simulink model "case6"  (R2024b)
settings: Solver=FixedStepAuto  StartTime=0  StopTime=1  FixedStep=1e-7  RelTol=1e-3
values from neighbouring files (symbols this model uses):
  SG_D_1_D = 0.01056    [IEEE9_case_parameters.m]    (also in case1_parameters.m; case2_parameters.m; case3_parameters.m; case4_parameters.m)
  SG_D_1_EnableSaturation = 0    [IEEE9_case_parameters.m]    (also in case1_parameters.m; case2_parameters.m; case3_parameters.m; case4_parameters.m)
  SG_D_1_f0 = 60    [IEEE9_case_parameters.m]    (also in case1_parameters.m; case2_parameters.m; case3_parameters.m; case4_parameters.m)
  SG_D_1_H = 7.5    [IEEE9_case_parameters.m]    (also in case1_parameters.m; case2_parameters.m; case3_parameters.m; case4_parameters.m)
  SG_D_1_K_A = 20    [IEEE9_case_parameters.m]    (also in case1_parameters.m; case2_parameters.m; case3_parameters.m; case4_parameters.m)
  SG_D_1_K_E = 1.000000e+1    (= 10)    [IEEE9_case_parameters.m]    (also in case1_parameters.m; case2_parameters.m; case3_parameters.m; case4_parameters.m)
  SG_D_1_K_F = 2.363    [IEEE9_case_parameters.m]    (also in case1_parameters.m; case2_parameters.m; case3_parameters.m; case4_parameters.m)
  SG_D_1_K_s = 0.5    [IEEE9_case_parameters.m]    (also in case1_parameters.m = 5; case2_parameters.m = 5; case3_parameters.m = 5; case4_parameters.m = 5)
  SG_D_1_R_a = 0.001088    [IEEE9_case_parameters.m]    (also in case1_parameters.m; case2_parameters.m; case3_parameters.m; case4_parameters.m)
  SG_D_1_S_A = 1    [IEEE9_case_parameters.m]    (also in case1_parameters.m; case2_parameters.m; case3_parameters.m; case4_parameters.m)
  SG_D_1_S_B = 0.103    [IEEE9_case_parameters.m]    (also in case1_parameters.m; case2_parameters.m; case3_parameters.m; case4_parameters.m)
  SG_D_1_S_N = 10.659857    [IEEE9_case_parameters.m]    (also in case1_parameters.m; case2_parameters.m; case3_parameters.m; case4_parameters.m)
  SG_D_1_SpeedPara = 200    [IEEE9_case_parameters.m]    (also in case1_parameters.m; case2_parameters.m; case3_parameters.m; case4_parameters.m)
  SG_D_1_T_0 = 0.720173    [IEEE9_case_parameters.m]    (also in case1_parameters.m = 0.755522; case2_parameters.m = 0.808931; case3_parameters.m = 0.869402; case4_parameters.m = 0.729316)
  SG_D_1_T_1 = 0.3    [IEEE9_case_parameters.m]    (also in case1_parameters.m; case2_parameters.m; case3_parameters.m; case4_parameters.m)
  SG_D_1_T_2 = 0.05    [IEEE9_case_parameters.m]    (also in case1_parameters.m; case2_parameters.m; case3_parameters.m; case4_parameters.m)
  SG_D_1_T_3 = 0.02    [IEEE9_case_parameters.m]    (also in case1_parameters.m; case2_parameters.m; case3_parameters.m; case4_parameters.m)
  SG_D_1_T_4 = 0.005    [IEEE9_case_parameters.m]    (also in case1_parameters.m; case2_parameters.m; case3_parameters.m; case4_parameters.m)
  SG_D_1_T_A = 0.02    [IEEE9_case_parameters.m]    (also in case1_parameters.m; case2_parameters.m; case3_parameters.m; case4_parameters.m)
  SG_D_1_T_dd = 8.000000e+0    (= 8)    [IEEE9_case_parameters.m]    (also in case1_parameters.m; case2_parameters.m; case3_parameters.m; case4_parameters.m)
  SG_D_1_T_ddd = 0.04    [IEEE9_case_parameters.m]    (also in case1_parameters.m; case2_parameters.m; case3_parameters.m; case4_parameters.m)
  SG_D_1_T_E = 0.314    [IEEE9_case_parameters.m]    (also in case1_parameters.m; case2_parameters.m; case3_parameters.m; case4_parameters.m)
  SG_D_1_T_F = 0.35    [IEEE9_case_parameters.m]    (also in case1_parameters.m; case2_parameters.m; case3_parameters.m; case4_parameters.m)
  SG_D_1_T_qd = 0.8    [IEEE9_case_parameters.m]    (also in case1_parameters.m; case2_parameters.m; case3_parameters.m; case4_parameters.m)
  SG_D_1_T_qdd = 0.02    [IEEE9_case_parameters.m]    (also in case1_parameters.m; case2_parameters.m; case3_parameters.m; case4_parameters.m)
  SG_D_1_T_speed = 0.1    [IEEE9_case_parameters.m]    (also in case1_parameters.m = 200; case2_parameters.m = 200; case3_parameters.m = 200; case4_parameters.m = 200)
  SG_D_1_T_w = 0.5    [IEEE9_case_parameters.m]    (also in case1_parameters.m; case2_parameters.m; case3_parameters.m; case4_parameters.m)
  SG_D_1_V_ref = 1.990276    [IEEE9_case_parameters.m]    (also in case1_parameters.m = 2.042296; case2_parameters.m = 2.051388; case3_parameters.m = 2.089584; case4_parameters.m = 2.01845)
  SG_D_1_w_ref = 376.991118    [IEEE9_case_parameters.m]    (also in case1_parameters.m; case2_parameters.m; case3_parameters.m; case4_parameters.m)
  SG_D_1_wb = 6.000000e+1    (= 60)    [IEEE9_case_parameters.m]    (also in case1_parameters.m; case2_parameters.m; case3_parameters.m; case4_parameters.m)
  SG_D_1_x_d = 1.9    [IEEE9_case_parameters.m]    (also in case1_parameters.m; case2_parameters.m; case3_parameters.m; case4_parameters.m)
  SG_D_1_x_dd = 0.302    [IEEE9_case_parameters.m]    (also in case1_parameters.m; case2_parameters.m; case3_parameters.m; case4_parameters.m)
  SG_D_1_x_ddd = 0.204    [IEEE9_case_parameters.m]    (also in case1_parameters.m; case2_parameters.m; case3_parameters.m; case4_parameters.m)
  SG_D_1_x_l = 0.05    [IEEE9_case_parameters.m]    (also in case1_parameters.m; case2_parameters.m; case3_parameters.m; case4_parameters.m)
  SG_D_1_x_q = 1.3    [IEEE9_case_parameters.m]    (also in case1_parameters.m; case2_parameters.m; case3_parameters.m; case4_parameters.m)
  SG_D_1_x_qd = 0.5    [IEEE9_case_parameters.m]    (also in case1_parameters.m; case2_parameters.m; case3_parameters.m; case4_parameters.m)
  SG_D_1_x_qdd = 0.3    [IEEE9_case_parameters.m]    (also in case1_parameters.m; case2_parameters.m; case3_parameters.m; case4_parameters.m)
  SG_D_2_D = 0.02    [IEEE9_case_parameters.m]    (also in case1_parameters.m; case2_parameters.m; case3_parameters.m; case4_parameters.m)
  SG_D_2_EnableSaturation = 0    [IEEE9_case_parameters.m]    (also in case1_parameters.m; case2_parameters.m; case3_parameters.m; case4_parameters.m)
  SG_D_2_f0 = 60    [IEEE9_case_parameters.m]    (also in case1_parameters.m; case2_parameters.m; case3_parameters.m; case4_parameters.m)
  SG_D_2_H = 8.000000e+0    (= 8)    [IEEE9_case_parameters.m]    (also in case1_parameters.m; case2_parameters.m; case3_parameters.m; case4_parameters.m)
  SG_D_2_K_A = 20    [IEEE9_case_parameters.m]    (also in case1_parameters.m; case2_parameters.m; case3_parameters.m; case4_parameters.m)
  SG_D_2_K_E = 1.000000e+1    (= 10)    [IEEE9_case_parameters.m]    (also in case1_parameters.m; case2_parameters.m; case3_parameters.m; case4_parameters.m)
  SG_D_2_K_F = 2.363    [IEEE9_case_parameters.m]    (also in case1_parameters.m; case2_parameters.m; case3_parameters.m; case4_parameters.m)
  SG_D_2_K_s = 0.5    [IEEE9_case_parameters.m]    (also in case1_parameters.m = 4; case2_parameters.m = 4; case3_parameters.m = 4; case4_parameters.m = 4)
  SG_D_2_R_a = 0.001088    [IEEE9_case_parameters.m]    (also in case1_parameters.m; case2_parameters.m; case3_parameters.m; case4_parameters.m)
  SG_D_2_S_A = 1    [IEEE9_case_parameters.m]    (also in case1_parameters.m; case2_parameters.m; case3_parameters.m; case4_parameters.m)
  SG_D_2_S_B = 0.103    [IEEE9_case_parameters.m]    (also in case1_parameters.m; case2_parameters.m; case3_parameters.m; case4_parameters.m)
  SG_D_2_S_N = 10.659857    [IEEE9_case_parameters.m]    (also in case1_parameters.m; case2_parameters.m; case3_parameters.m; case4_parameters.m)
  SG_D_2_SpeedPara = 200    [IEEE9_case_parameters.m]    (also in case1_parameters.m; case2_parameters.m; case3_parameters.m; case4_parameters.m)
  SG_D_2_T_0 = 1.632913    [IEEE9_case_parameters.m]    (also in case1_parameters.m = 1.632925; case2_parameters.m = 1.632915; case3_parameters.m = 1.632914; case4_parameters.m = 1.632927)
  SG_D_2_T_1 = 0.2    [IEEE9_case_parameters.m]    (also in case1_parameters.m; case2_parameters.m; case3_parameters.m; case4_parameters.m)
  SG_D_2_T_2 = 0.05    [IEEE9_case_parameters.m]    (also in case1_parameters.m; case2_parameters.m; case3_parameters.m; case4_parameters.m)
  SG_D_2_T_3 = 0.02    [IEEE9_case_parameters.m]    (also in case1_parameters.m; case2_parameters.m; case3_parameters.m; case4_parameters.m)
  SG_D_2_T_4 = 0.005    [IEEE9_case_parameters.m]    (also in case1_parameters.m; case2_parameters.m; case3_parameters.m; case4_parameters.m)
  SG_D_2_T_A = 0.02    [IEEE9_case_parameters.m]    (also in case1_parameters.m; case2_parameters.m; case3_parameters.m; case4_parameters.m)
  SG_D_2_T_dd = 7.9    [IEEE9_case_parameters.m]    (also in case1_parameters.m; case2_parameters.m; case3_parameters.m; case4_parameters.m)
  SG_D_2_T_ddd = 0.04    [IEEE9_case_parameters.m]    (also in case1_parameters.m; case2_parameters.m; case3_parameters.m; case4_parameters.m)
  SG_D_2_T_E = 0.314    [IEEE9_case_parameters.m]    (also in case1_parameters.m; case2_parameters.m; case3_parameters.m; case4_parameters.m)
  SG_D_2_T_F = 0.35    [IEEE9_case_parameters.m]    (also in case1_parameters.m; case2_parameters.m; case3_parameters.m; case4_parameters.m)
  SG_D_2_T_qd = 0.8    [IEEE9_case_parameters.m]    (also in case1_parameters.m; case2_parameters.m; case3_parameters.m; case4_parameters.m)
  SG_D_2_T_qdd = 0.015    [IEEE9_case_parameters.m]    (also in case1_parameters.m; case2_parameters.m; case3_parameters.m; case4_parameters.m)
  SG_D_2_T_speed = 0.1    [IEEE9_case_parameters.m]    (also in case1_parameters.m = 150; case2_parameters.m = 150; case3_parameters.m = 150; case4_parameters.m = 150)
  SG_D_2_T_w = 0.35    [IEEE9_case_parameters.m]    (also in case1_parameters.m; case2_parameters.m; case3_parameters.m; case4_parameters.m)
  SG_D_2_V_ref = 2.58547    [IEEE9_case_parameters.m]    (also in case1_parameters.m = 2.597896; case2_parameters.m = 2.587136; case3_parameters.m = 2.586042; case4_parameters.m = 2.599679)
  SG_D_2_w_ref = 376.991118    [IEEE9_case_parameters.m]    (also in case1_parameters.m; case2_parameters.m; case3_parameters.m; case4_parameters.m)
  SG_D_2_wb = 6.000000e+1    (= 60)    [IEEE9_case_parameters.m]    (also in case1_parameters.m; case2_parameters.m; case3_parameters.m; case4_parameters.m)
  SG_D_2_x_d = 1.8    [IEEE9_case_parameters.m]    (also in case1_parameters.m; case2_parameters.m; case3_parameters.m; case4_parameters.m)
  SG_D_2_x_dd = 0.302    [IEEE9_case_parameters.m]    (also in case1_parameters.m; case2_parameters.m; case3_parameters.m; case4_parameters.m)
  SG_D_2_x_ddd = 0.204    [IEEE9_case_parameters.m]    (also in case1_parameters.m; case2_parameters.m; case3_parameters.m; case4_parameters.m)
  SG_D_2_x_l = 0.05    [IEEE9_case_parameters.m]    (also in case1_parameters.m; case2_parameters.m; case3_parameters.m; case4_parameters.m)
  SG_D_2_x_q = 1.25    [IEEE9_case_parameters.m]    (also in case1_parameters.m; case2_parameters.m; case3_parameters.m; case4_parameters.m)
  SG_D_2_x_qd = 0.5    [IEEE9_case_parameters.m]    (also in case1_parameters.m; case2_parameters.m; case3_parameters.m; case4_parameters.m)
  SG_D_2_x_qdd = 0.3    [IEEE9_case_parameters.m]    (also in case1_parameters.m; case2_parameters.m; case3_parameters.m; case4_parameters.m)
  SG_D_3_D = 0.02    [IEEE9_case_parameters.m]    (also in case1_parameters.m; case2_parameters.m; case3_parameters.m; case4_parameters.m)
  SG_D_3_EnableSaturation = 0    [IEEE9_case_parameters.m]    (also in case1_parameters.m; case2_parameters.m; case3_parameters.m; case4_parameters.m)
  SG_D_3_f0 = 60    [IEEE9_case_parameters.m]    (also in case1_parameters.m; case2_parameters.m; case3_parameters.m; case4_parameters.m)
  SG_D_3_H = 7.7    [IEEE9_case_parameters.m]    (also in case1_parameters.m; case2_parameters.m; case3_parameters.m; case4_parameters.m)
  SG_D_3_K_A = 20    [IEEE9_case_parameters.m]    (also in case1_parameters.m; case2_parameters.m; case3_parameters.m; case4_parameters.m)
  SG_D_3_K_E = 1.000000e+1    (= 10)    [IEEE9_case_parameters.m]    (also in case1_parameters.m; case2_parameters.m; case3_parameters.m; case4_parameters.m)
  SG_D_3_K_F = 2.363    [IEEE9_case_parameters.m]    (also in case1_parameters.m; case2_parameters.m; case3_parameters.m; case4_parameters.m)
  SG_D_3_K_s = 0.2    [IEEE9_case_parameters.m]    (also in case1_parameters.m = 2; case2_parameters.m = 2; case3_parameters.m = 2; case4_parameters.m = 2)
  SG_D_3_R_a = 0.001088    [IEEE9_case_parameters.m]    (also in case1_parameters.m; case2_parameters.m; case3_parameters.m; case4_parameters.m)
  SG_D_3_S_A = 1    [IEEE9_case_parameters.m]    (also in case1_parameters.m; case2_parameters.m; case3_parameters.m; case4_parameters.m)
  SG_D_3_S_B = 0.103    [IEEE9_case_parameters.m]    (also in case1_parameters.m; case2_parameters.m; case3_parameters.m; case4_parameters.m)
  SG_D_3_S_N = 10.659857    [IEEE9_case_parameters.m]    (also in case1_parameters.m; case2_parameters.m; case3_parameters.m; case4_parameters.m)
  SG_D_3_SpeedPara = 200    [IEEE9_case_parameters.m]    (also in case1_parameters.m; case2_parameters.m; case3_parameters.m; case4_parameters.m)
  SG_D_3_T_0 = 0.850788    [IEEE9_case_parameters.m]    (also in case1_parameters.m = 0.850786; case2_parameters.m = 0.850787; case3_parameters.m; case4_parameters.m = 0.850786)
  SG_D_3_T_1 = 0.2    [IEEE9_case_parameters.m]    (also in case1_parameters.m; case2_parameters.m; case3_parameters.m; case4_parameters.m)
  SG_D_3_T_2 = 0.05    [IEEE9_case_parameters.m]    (also in case1_parameters.m; case2_parameters.m; case3_parameters.m; case4_parameters.m)
  SG_D_3_T_3 = 0.02    [IEEE9_case_parameters.m]    (also in case1_parameters.m; case2_parameters.m; case3_parameters.m; case4_parameters.m)
  SG_D_3_T_4 = 0.005    [IEEE9_case_parameters.m]    (also in case1_parameters.m; case2_parameters.m; case3_parameters.m; case4_parameters.m)
  SG_D_3_T_A = 0.02    [IEEE9_case_parameters.m]    (also in case1_parameters.m; case2_parameters.m; case3_parameters.m; case4_parameters.m)
  SG_D_3_T_dd = 8.1    [IEEE9_case_parameters.m]    (also in case1_parameters.m; case2_parameters.m; case3_parameters.m; case4_parameters.m)
  SG_D_3_T_ddd = 0.04    [IEEE9_case_parameters.m]    (also in case1_parameters.m; case2_parameters.m; case3_parameters.m; case4_parameters.m)
  SG_D_3_T_E = 0.314    [IEEE9_case_parameters.m]    (also in case1_parameters.m; case2_parameters.m; case3_parameters.m; case4_parameters.m)
  SG_D_3_T_F = 0.35    [IEEE9_case_parameters.m]    (also in case1_parameters.m; case2_parameters.m; case3_parameters.m; case4_parameters.m)
  SG_D_3_T_qd = 0.8    [IEEE9_case_parameters.m]    (also in case1_parameters.m; case2_parameters.m; case3_parameters.m; case4_parameters.m)
  SG_D_3_T_qdd = 0.015    [IEEE9_case_parameters.m]    (also in case1_parameters.m; case2_parameters.m; case3_parameters.m; case4_parameters.m)
  SG_D_3_T_speed = 0.1    [IEEE9_case_parameters.m]    (also in case1_parameters.m = 180; case2_parameters.m = 180; case3_parameters.m = 180; case4_parameters.m = 180)
  SG_D_3_T_w = 0.4    [IEEE9_case_parameters.m]    (also in case1_parameters.m; case2_parameters.m; case3_parameters.m; case4_parameters.m)
  SG_D_3_V_ref = 1.892727    [IEEE9_case_parameters.m]    (also in case1_parameters.m = 1.906439; case2_parameters.m = 1.895535; case3_parameters.m = 1.892105; case4_parameters.m = 1.906598)
  SG_D_3_w_ref = 376.991118    [IEEE9_case_parameters.m]    (also in case1_parameters.m; case2_parameters.m; case3_parameters.m; case4_parameters.m)
  SG_D_3_wb = 6.000000e+1    (= 60)    [IEEE9_case_parameters.m]    (also in case1_parameters.m; case2_parameters.m; case3_parameters.m; case4_parameters.m)
  SG_D_3_x_d = 1.85    [IEEE9_case_parameters.m]    (also in case1_parameters.m; case2_parameters.m; case3_parameters.m; case4_parameters.m)
  SG_D_3_x_dd = 0.302    [IEEE9_case_parameters.m]    (also in case1_parameters.m; case2_parameters.m; case3_parameters.m; case4_parameters.m)
  SG_D_3_x_ddd = 0.204    [IEEE9_case_parameters.m]    (also in case1_parameters.m; case2_parameters.m; case3_parameters.m; case4_parameters.m)
  SG_D_3_x_l = 0.05    [IEEE9_case_parameters.m]    (also in case1_parameters.m; case2_parameters.m; case3_parameters.m; case4_parameters.m)
  SG_D_3_x_q = 1.2    [IEEE9_case_parameters.m]    (also in case1_parameters.m; case2_parameters.m; case3_parameters.m; case4_parameters.m)
  SG_D_3_x_qd = 0.5    [IEEE9_case_parameters.m]    (also in case1_parameters.m; case2_parameters.m; case3_parameters.m; case4_parameters.m)
  SG_D_3_x_qdd = 0.3    [IEEE9_case_parameters.m]    (also in case1_parameters.m; case2_parameters.m; case3_parameters.m; case4_parameters.m)
(part 6 of 12)

== system case6/SG_D_1/d_psi_kq_SG_D_1_block ==
  note: d_psi_kq_SG_D_1 in case6
      | $-\frac{\psi _{\mathrm{gq},\mathrm{SG},D,1}+\psi _{\mathrm{kq},\mathrm{SG},D,1}+\frac{\left(x_{l}-x_{\mathrm{qd}}\right)\,\left(\psi _{q,\mathrm{SG},D,1}+\frac{\psi _{\mathrm{gq},\mathrm{SG},D,1}\,\left(x_{l}-x_{\mathrm{qdd}}\right)}{x_{l}-x_{\mathrm{qd}}}+\frac{\psi _{\mathrm{kq},\mathrm{SG},D,1}\,\left(x_{\mathrm{qd}}-x_{\mathrm{qdd}}\right)}{x_{l}-x_{\mathrm{qd}}}\right)}{x_{\mathrm{qdd}}}}{T_{\mathrm{qdd}}}$
      | Automatically generated on 2025-10-31 19:16:47 .
  State_psi_gq_SG_D_1_a2f76 : Inport
  State_psi_kq_SG_D_1_0796b : Inport  Port=2
  State_psi_gq_SG_D_1_98e41 : Inport  Port=3
  State_psi_kq_SG_D_1_e206f : Inport  Port=4
  State_psi_q_SG_D_1_2866b : Inport  Port=5
  Add_1a6d4 : Sum
  Add_1c684 : Sum
  Add_23d6a : Sum
  Add_3dcaa : Sum
  Add_3fd01 : Sum
  Add_ae08e : Sum
  Constant_-1_30ef9 : Constant  Value=-1
  Constant_-1_38b5b : Constant  Value=-1
  Constant_-1_7cc70 : Constant  Value=-1
  Constant_-1_86c96 : Constant  Value=-1
  Constant_-1_87d0c : Constant  Value=-1
  Constant_T_qdd_6ced7 : Constant  Value=T_qdd
  Constant_x_l_74132 : Constant  Value=x_l
  Constant_x_l_a1695 : Constant  Value=x_l
  Constant_x_l_cfba1 : Constant  Value=x_l
  Constant_x_l_dd985 : Constant  Value=x_l
  Constant_x_qd_677a7 : Constant  Value=x_qd
  Constant_x_qd_7f0f9 : Constant  Value=x_qd
  Constant_x_qd_c83dc : Constant  Value=x_qd
  Constant_x_qd_fa9ab : Constant  Value=x_qd
  Constant_x_qdd_32a72 : Constant  Value=x_qdd
  Constant_x_qdd_ea146 : Constant  Value=x_qdd
  Constant_x_qdd_ef1b3 : Constant  Value=x_qdd
  Divide_06d40 : Product  Inputs=*/
  Divide_5f361 : Product  Inputs=*/
  Divide_6ce48 : Product  Inputs=*/
  Divide_87f21 : Product  Inputs=*/
  Product_14234 : Product
  Product_395bf : Product
  Product_63ba5 : Product
  Product_6528f : Product
  Product_a4f2e : Product
  Product_a7cd9 : Product
  Product_e18f5 : Product
  Product_fddf8 : Product
  Subtract_18d5b : Sum  Inputs=+-
  Subtract_82111 : Sum  Inputs=+-
  Subtract_f6316 : Sum  Inputs=+-
  Blockout_d_psi_kq_SG_D_1_a926e : Outport
  wires:
  Product_6528f/1 -> Add_23d6a/1
  Constant_-1_38b5b/1 -> Product_6528f/1
  Constant_x_l_74132/1 -> Product_6528f/2
  Constant_x_qdd_ef1b3/1 -> Add_23d6a/2
  Constant_-1_87d0c/1 -> Product_e18f5/1
  Constant_x_qd_7f0f9/1 -> Subtract_f6316/1
  Constant_x_qd_c83dc/1 -> Add_1c684/2
  Constant_-1_30ef9/1 -> Product_a7cd9/1
  Constant_x_l_dd985/1 -> Product_e18f5/2
  Constant_x_qdd_32a72/1 -> Subtract_f6316/2
  Constant_x_qd_677a7/1 -> Add_ae08e/2
  Constant_x_l_a1695/1 -> Product_a7cd9/2
  Subtract_82111/1 -> Add_1a6d4/1
  Product_395bf/1 -> Subtract_82111/1
  State_psi_gq_SG_D_1_98e41/1 -> Product_63ba5/1
  Add_23d6a/1 -> Product_63ba5/2
  Product_a7cd9/1 -> Add_3fd01/1
  Constant_x_qd_fa9ab/1 -> Add_3fd01/2
  State_psi_kq_SG_D_1_e206f/1 -> Product_14234/1
  Product_e18f5/1 -> Add_ae08e/1
  Subtract_f6316/1 -> Product_14234/2
  Product_63ba5/1 -> Divide_6ce48/1
  Add_3fd01/1 -> Divide_6ce48/2
  Product_14234/1 -> Divide_5f361/1
  Add_ae08e/1 -> Divide_5f361/2
  Constant_-1_7cc70/1 -> Product_a4f2e/1
  Constant_x_l_cfba1/1 -> Product_a4f2e/2
  Divide_6ce48/1 -> Subtract_18d5b/1
  Divide_5f361/1 -> Subtract_18d5b/2
  Product_a4f2e/1 -> Add_1c684/1
  Add_3dcaa/1 -> Product_fddf8/2
  Subtract_18d5b/1 -> Add_3dcaa/1
  State_psi_q_SG_D_1_2866b/1 -> Add_3dcaa/2
  Constant_-1_86c96/1 -> Product_395bf/1
  State_psi_gq_SG_D_1_a2f76/1 -> Product_395bf/2
  Divide_06d40/1 -> Add_1a6d4/2
  Product_fddf8/1 -> Divide_06d40/1
  Add_1c684/1 -> Product_fddf8/1
  State_psi_kq_SG_D_1_0796b/1 -> Subtract_82111/2
  Constant_x_qdd_ea146/1 -> Divide_06d40/2
  Add_1a6d4/1 -> Divide_87f21/1
  Constant_T_qdd_6ced7/1 -> Divide_87f21/2
  Divide_87f21/1 -> Blockout_d_psi_kq_SG_D_1_a926e/1

== system case6/SG_D_1/d_psi_q_SG_D_1_block ==
  note: d_psi_q_SG_D_1 in case6
      | $2\,\pi \,f_{0}\,\left(v_{d,\mathrm{SG},D,1}\,\cos\left(\theta _{\mathrm{SG},D,1}\right)+v_{q,\mathrm{SG},D,1}\,\sin\left(\theta _{\mathrm{SG},D,1}\right)-\frac{R_{a}\,\left(\psi _{q,\mathrm{SG},D,1}+\frac{\psi _{\mathrm{gq},\mathrm{SG},D,1}\,\left(x_{l}-x_{\mathrm{qdd}}\right)}{x_{l}-x_{\mathrm{qd}}}+\frac{\psi _{\mathrm{kq},\mathrm{SG},D,1}\,\left(x_{\mathrm{qd}}-x_{\mathrm{qdd}}\right)}{x_{l}-x_{\mathrm{qd}}}\right)}{x_{\mathrm{qdd}}}-\frac{\psi _{d,\mathrm{SG},D,1}\,w_{\mathrm{SG},D,1}}{2\,f_{0}\,\pi }\right)$
      | Automatically generated on 2025-10-31 19:16:30 .
  State_psi_gq_SG_D_1_ab6b9 : Inport
  State_psi_kq_SG_D_1_59706 : Inport  Port=2
  State_psi_q_SG_D_1_a6dfc : Inport  Port=3
  Input_v_d_SG_D_1_0ed7f : Inport  Port=4
  State_theta_SG_D_1_d9d3f : Inport  Port=5
  Input_v_q_SG_D_1_06492 : Inport  Port=6
  State_theta_SG_D_1_9a223 : Inport  Port=7
  State_psi_d_SG_D_1_bfedb : Inport  Port=8
  State_w_SG_D_1_c3b6c : Inport  Port=9
  Add_5280d : Sum
  Add_61884 : Sum
  Add_80cdb : Sum
  Add_c7e31 : Sum
  Add_f9285 : Sum
  Constant_-1_3b70b : Constant  Value=-1
  Constant_-1_682dd : Constant  Value=-1
  Constant_-1_6cf58 : Constant  Value=-1
  Constant_-2.0_91d52 : Constant  Value=-2.0
  Constant_2.0_f8821 : Constant  Value=2.0
  Constant_R_a_f62d9 : Constant  Value=R_a
  Constant_f0_7f90b : Constant  Value=f0
  Constant_f0_f6419 : Constant  Value=f0
  Constant_pi_0eb2d : Constant  Value=pi
  Constant_pi_c72a0 : Constant  Value=pi
  Constant_x_l_02cf9 : Constant  Value=x_l
  Constant_x_l_3bcf4 : Constant  Value=x_l
  Constant_x_l_46b1e : Constant  Value=x_l
  Constant_x_qd_06e65 : Constant  Value=x_qd
  Constant_x_qd_5b463 : Constant  Value=x_qd
  Constant_x_qd_63e08 : Constant  Value=x_qd
  Constant_x_qdd_27940 : Constant  Value=x_qdd
  Constant_x_qdd_a542f : Constant  Value=x_qdd
  Constant_x_qdd_c014d : Constant  Value=x_qdd
  Divide_100b8 : Product  Inputs=*/
  Divide_13002 : Product  Inputs=*/
  Divide_88f3a : Product  Inputs=*/
  Divide_89af9 : Product  Inputs=*/
  MathFunc_cos_75e4d : Trigonometry  Operator=cos
  MathFunc_sin_b6dca : Trigonometry
  Product_1b7d0 : Product
  Product_3d15a : Product
  Product_5f438 : Product
  Product_80704 : Product
  Product_88a91 : Product
  Product_a56d1 : Product
  Product_af8c6 : Product
  Product_b585f : Product
  Product_c04a9 : Product
  Product_dc704 : Product
  Product_e4fa3 : Product
  Product_ec679 : Product
  Product_ecac2 : Product
  Product_fdb14 : Product
  Subtract_8d5ad : Sum  Inputs=+-
  Subtract_c7687 : Sum  Inputs=+-
  Subtract_d1877 : Sum  Inputs=+-
  Subtract_e85cf : Sum  Inputs=+-
  Blockout_d_psi_q_SG_D_1_6a810 : Outport
  wires:
  Divide_100b8/1 -> Subtract_8d5ad/1
  Product_c04a9/1 -> Add_c7e31/1
  Constant_x_l_46b1e/1 -> Product_c04a9/2
  Constant_-1_3b70b/1 -> Product_c04a9/1
  Constant_x_qdd_27940/1 -> Add_c7e31/2
  Constant_x_l_02cf9/1 -> Product_ec679/2
  Constant_-1_6cf58/1 -> Product_ec679/1
  Constant_x_l_3bcf4/1 -> Product_1b7d0/2
  Constant_x_qdd_c014d/1 -> Subtract_c7687/2
  State_psi_kq_SG_D_1_59706/1 -> Product_80704/1
  Constant_-1_682dd/1 -> Product_1b7d0/1
  Constant_x_qd_06e65/1 -> Subtract_c7687/1
  State_psi_gq_SG_D_1_ab6b9/1 -> Product_af8c6/1
  Product_fdb14/1 -> Blockout_d_psi_q_SG_D_1_6a810/1
  Subtract_8d5ad/1 -> Add_f9285/1
  Product_af8c6/1 -> Divide_100b8/1
  Add_c7e31/1 -> Product_af8c6/2
  Divide_88f3a/1 -> Subtract_8d5ad/2
  Product_ec679/1 -> Add_5280d/1
  Constant_x_qd_63e08/1 -> Add_5280d/2
  Constant_-2.0_91d52/1 -> Product_a56d1/1
  Product_80704/1 -> Divide_88f3a/1
  Product_1b7d0/1 -> Add_61884/1
  Subtract_c7687/1 -> Product_80704/2
  Constant_x_qd_5b463/1 -> Add_61884/2
  Add_5280d/1 -> Divide_100b8/2
  Add_61884/1 -> Divide_88f3a/2
  Constant_f0_7f90b/1 -> Product_ecac2/2
  State_psi_q_SG_D_1_a6dfc/1 -> Add_f9285/2
  Product_e4fa3/1 -> Product_b585f/1
  Constant_R_a_f62d9/1 -> Product_dc704/1
  Product_b585f/1 -> Divide_13002/2
  Product_dc704/1 -> Divide_89af9/1
  Add_f9285/1 -> Product_dc704/2
  State_theta_SG_D_1_d9d3f/1 -> MathFunc_cos_75e4d/1
  Input_v_d_SG_D_1_0ed7f/1 -> Product_5f438/1
  Constant_x_qdd_a542f/1 -> Divide_89af9/2
  MathFunc_cos_75e4d/1 -> Product_5f438/2
  State_theta_SG_D_1_9a223/1 -> MathFunc_sin_b6dca/1
  Divide_89af9/1 -> Subtract_e85cf/1
  Constant_2.0_f8821/1 -> Product_e4fa3/1
  State_w_SG_D_1_c3b6c/1 -> Product_88a91/2
  Constant_pi_0eb2d/1 -> Product_e4fa3/2
  Subtract_d1877/1 -> Add_80cdb/1
  Product_5f438/1 -> Subtract_e85cf/2
  Divide_13002/1 -> Add_80cdb/2
  Input_v_q_SG_D_1_06492/1 -> Product_3d15a/1
  MathFunc_sin_b6dca/1 -> Product_3d15a/2
  Product_3d15a/1 -> Subtract_d1877/2
  State_psi_d_SG_D_1_bfedb/1 -> Product_88a91/1
  Constant_f0_f6419/1 -> Product_b585f/2
  Constant_pi_c72a0/1 -> Product_a56d1/2
  Subtract_e85cf/1 -> Subtract_d1877/1
  Product_88a91/1 -> Divide_13002/1
  Product_a56d1/1 -> Product_ecac2/1
  Product_ecac2/1 -> Product_fdb14/1
  Add_80cdb/1 -> Product_fdb14/2

== system case6/SG_D_1/d_theta_SG_D_1_block ==
  note: d_theta_SG_D_1 in case6
      | $w_{\mathrm{SG},D,1}-2\,\pi \,f_{0}$
      | Automatically generated on 2025-10-31 19:16:54 .
  State_w_SG_D_1_0521f : Inport
  Add_4df2e : Sum
  Constant_-2.0_50b2e : Constant  Value=-2.0
  Constant_f0_88e41 : Constant  Value=f0
  Constant_pi_90045 : Constant  Value=pi
  Product_29839 : Product
  Product_44238 : Product
  Blockout_d_theta_SG_D_1_90efe : Outport
  wires:
  State_w_SG_D_1_0521f/1 -> Add_4df2e/2
  Constant_-2.0_50b2e/1 -> Product_44238/1
  Constant_f0_88e41/1 -> Product_29839/2
  Constant_pi_90045/1 -> Product_44238/2
  Product_29839/1 -> Add_4df2e/1
  Product_44238/1 -> Product_29839/1
  Add_4df2e/1 -> Blockout_d_theta_SG_D_1_90efe/1

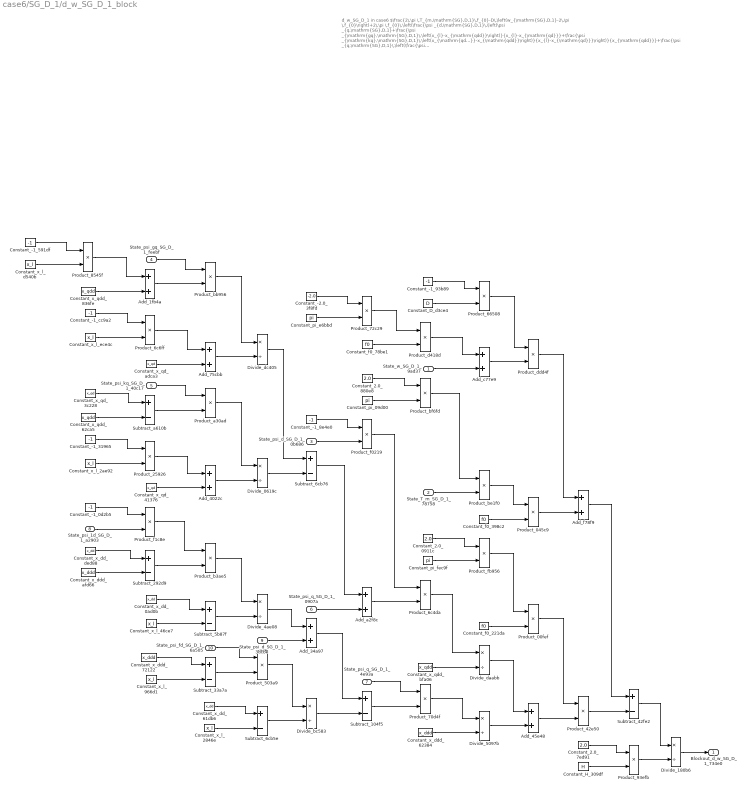
== system case6/SG_D_1/d_w_SG_D_1_block ==
  note: d_w_SG_D_1 in case6
      | $\frac{2\,\pi \,T_{m,\mathrm{SG},D,1}\,f_{0}-D\,\left(w_{\mathrm{SG},D,1}-2\,\pi \,f_{0}\right)+2\,\pi \,f_{0}\,\left(\frac{\psi _{d,\mathrm{SG},D,1}\,\left(\psi _{q,\mathrm{SG},D,1}+\frac{\psi _{\mathrm{gq},\mathrm{SG},D,1}\,\left(x_{l}-x_{\mathrm{qdd}}\right)}{x_{l}-x_{\mathrm{qd}}}+\frac{\psi _{\mathrm{kq},\mathrm{SG},D,1}\,\left(x_{\mathrm{qd}}-x_{\mathrm{qdd}}\right)}{x_{l}-x_{\mathrm{qd}}}\right)}{x_{\mathrm{qdd}}}+\frac{\psi _{q,\mathrm{SG},D,1}\,\left(\frac{\psi _{\mathrm{1d},\mathrm{SG},D,1}\,\left(x_{\mathrm{dd}}-x_{\mathrm{ddd}}\right)}{x_{\mathrm{dd}}-x_{l}}-\psi _{d,\mathrm{SG},D,1}+\frac{\psi _{\mathrm{fd},\mathrm{SG},D,1}\,\left(x_{\mathrm{ddd}}-x_{l}\right)}{x_{\mathrm{dd}}-x_{l}}\right)}{x_{\mathrm{ddd}}}\right)}{2\,H}$
      | Automatically generated on 2025-10-31 19:16:52 .
  State_w_SG_D_1_9ad37 : Inport
  State_T_m_SG_D_1_78758 : Inport  Port=2
  State_psi_d_SG_D_1_0b686 : Inport  Port=3
  State_psi_gq_SG_D_1_feebf : Inport  Port=4
  State_psi_kq_SG_D_1_40c17 : Inport  Port=5
  State_psi_q_SG_D_1_0907a : Inport  Port=6
  State_psi_q_SG_D_1_4e93a : Inport  Port=7
  State_psi_1d_SG_D_1_a2903 : Inport  Port=8
  State_psi_d_SG_D_1_3dcbe : Inport  Port=9
  State_psi_fd_SG_D_1_6a505 : Inport  Port=10
  Add_1fb4a : Sum
  Add_34a97 : Sum
  Add_4022c : Sum
  Add_45e48 : Sum
  Add_75cbb : Sum
  Add_a2f8c : Sum
  Add_c77e9 : Sum
  Add_f78f9 : Sum
  Constant_-1_0d2b5 : Constant  Value=-1
  Constant_-1_31965 : Constant  Value=-1
  Constant_-1_591df : Constant  Value=-1
  Constant_-1_8e4e0 : Constant  Value=-1
  Constant_-1_93b89 : Constant  Value=-1
  Constant_-1_cc9a2 : Constant  Value=-1
  Constant_-2.0_3f8fd : Constant  Value=-2.0
  Constant_2.0_0911c : Constant  Value=2.0
  Constant_2.0_7ed91 : Constant  Value=2.0
  Constant_2.0_880e8 : Constant  Value=2.0
  Constant_D_d3ce4 : Constant  Value=D
  Constant_H_309df : Constant  Value=H
  Constant_f0_221da : Constant  Value=f0
  Constant_f0_398c2 : Constant  Value=f0
  Constant_f0_78be1 : Constant  Value=f0
  Constant_pi_09d00 : Constant  Value=pi
  Constant_pi_e6bbd : Constant  Value=pi
  Constant_pi_fec9f : Constant  Value=pi
  Constant_x_dd_0ad0b : Constant  Value=x_dd
  Constant_x_dd_61db6 : Constant  Value=x_dd
  Constant_x_dd_ded88 : Constant  Value=x_dd
  Constant_x_ddd_62384 : Constant  Value=x_ddd
  Constant_x_ddd_72122 : Constant  Value=x_ddd
  Constant_x_ddd_afd66 : Constant  Value=x_ddd
  Constant_x_l_2846e : Constant  Value=x_l
  Constant_x_l_2ae92 : Constant  Value=x_l
  Constant_x_l_46ce7 : Constant  Value=x_l
  Constant_x_l_966d1 : Constant  Value=x_l
  Constant_x_l_d540b : Constant  Value=x_l
  Constant_x_l_ece4c : Constant  Value=x_l
  Constant_x_qd_3c228 : Constant  Value=x_qd
  Constant_x_qd_41376 : Constant  Value=x_qd
  Constant_x_qd_adca3 : Constant  Value=x_qd
  Constant_x_qdd_62ca5 : Constant  Value=x_qdd
  Constant_x_qdd_836fe : Constant  Value=x_qdd
  Constant_x_qdd_bfa06 : Constant  Value=x_qdd
  Divide_0619c : Product  Inputs=*/
  Divide_180b6 : Product  Inputs=*/
  Divide_4ae08 : Product  Inputs=*/
  Divide_5097b : Product  Inputs=*/
  Divide_bc583 : Product  Inputs=*/
  Divide_daabb : Product  Inputs=*/
  Divide_dc405 : Product  Inputs=*/
  Product_00fef : Product
  Product_045c9 : Product
  Product_25926 : Product
  Product_42e50 : Product
  Product_503a9 : Product
  Product_66508 : Product
  Product_6c4da : Product
  Product_6c6ff : Product
  Product_70d4f : Product
  Product_72c29 : Product
  Product_8545f : Product
  Product_93efb : Product
  Product_a30ad : Product
  Product_b3ae5 : Product
  Product_bb956 : Product
  Product_be1f0 : Product
  Product_bf6fd : Product
  Product_d418d : Product
  Product_ddd4f : Product
  Product_f0219 : Product
  Product_f1c8e : Product
  Product_fb956 : Product
  Subtract_104f5 : Sum  Inputs=+-
  Subtract_292d9 : Sum  Inputs=+-
  Subtract_33a7a : Sum  Inputs=+-
  Subtract_42fe2 : Sum  Inputs=+-
  Subtract_5b87f : Sum  Inputs=+-
  Subtract_6cb5e : Sum  Inputs=+-
  Subtract_6cb76 : Sum  Inputs=+-
  Subtract_a610b : Sum  Inputs=+-
  Blockout_d_w_SG_D_1_734e0 : Outport
  wires:
  Product_d418d/1 -> Add_c77e9/1
  Constant_-1_591df/1 -> Product_8545f/1
  Constant_pi_09d00/1 -> Product_bf6fd/2
  Constant_x_qdd_836fe/1 -> Add_1fb4a/2
  Constant_x_l_d540b/1 -> Product_8545f/2
  Product_8545f/1 -> Add_1fb4a/1
  Constant_x_qd_3c228/1 -> Subtract_a610b/1
  Constant_-1_cc9a2/1 -> Product_6c6ff/1
  Product_72c29/1 -> Product_d418d/1
  Constant_x_qdd_62ca5/1 -> Subtract_a610b/2
  State_psi_q_SG_D_1_4e93a/1 -> Product_70d4f/1
  Constant_x_l_ece4c/1 -> Product_6c6ff/2
  Constant_-1_31965/1 -> Product_25926/1
  Constant_x_l_2ae92/1 -> Product_25926/2
  Constant_-1_0d2b5/1 -> Product_f1c8e/1
  Product_6c6ff/1 -> Add_75cbb/1
  State_psi_1d_SG_D_1_a2903/1 -> Product_f1c8e/2
  Constant_x_dd_ded88/1 -> Subtract_292d9/1
  Subtract_a610b/1 -> Product_a30ad/2
  Constant_x_ddd_afd66/1 -> Subtract_292d9/2
  State_psi_gq_SG_D_1_feebf/1 -> Product_bb956/1
  Product_f0219/1 -> Product_6c4da/1
  Add_1fb4a/1 -> Product_bb956/2
  Constant_x_qd_adca3/1 -> Add_75cbb/2
  State_psi_kq_SG_D_1_40c17/1 -> Product_a30ad/1
  Constant_f0_78be1/1 -> Product_d418d/2
  Product_25926/1 -> Add_4022c/1
  Constant_x_dd_0ad0b/1 -> Subtract_5b87f/1
  Constant_x_qd_41376/1 -> Add_4022c/2
  Product_f1c8e/1 -> Product_b3ae5/1
  Subtract_292d9/1 -> Product_b3ae5/2
  Constant_x_l_46ce7/1 -> Subtract_5b87f/2
  Constant_x_ddd_72122/1 -> Subtract_33a7a/1
  Constant_x_l_966d1/1 -> Subtract_33a7a/2
  State_w_SG_D_1_9ad37/1 -> Add_c77e9/2
  Divide_daabb/1 -> Add_45e48/1
  Constant_-1_93b89/1 -> Product_66508/1
  Product_bb956/1 -> Divide_dc405/1
  Add_c77e9/1 -> Product_ddd4f/2
  Divide_dc405/1 -> Subtract_6cb76/1
  Add_75cbb/1 -> Divide_dc405/2
  Constant_pi_e6bbd/1 -> Product_72c29/2
  Product_a30ad/1 -> Divide_0619c/1
  Add_4022c/1 -> Divide_0619c/2
  Product_b3ae5/1 -> Divide_4ae08/1
  Divide_4ae08/1 -> Add_34a97/1
  Subtract_5b87f/1 -> Divide_4ae08/2
  State_psi_fd_SG_D_1_6a505/1 -> Product_503a9/1
  Subtract_33a7a/1 -> Product_503a9/2
  Constant_x_dd_61db6/1 -> Subtract_6cb5e/1
  Constant_x_l_2846e/1 -> Subtract_6cb5e/2
  Divide_0619c/1 -> Subtract_6cb76/2
  Constant_2.0_880e8/1 -> Product_bf6fd/1
  State_psi_d_SG_D_1_3dcbe/1 -> Add_34a97/2
  Product_503a9/1 -> Divide_bc583/1
  Subtract_6cb5e/1 -> Divide_bc583/2
  Constant_-2.0_3f8fd/1 -> Product_72c29/1
  Constant_-1_8e4e0/1 -> Product_f0219/1
  State_psi_d_SG_D_1_0b686/1 -> Product_f0219/2
  Subtract_6cb76/1 -> Add_a2f8c/1
  Subtract_104f5/1 -> Product_70d4f/2
  State_psi_q_SG_D_1_0907a/1 -> Add_a2f8c/2
  Add_34a97/1 -> Subtract_104f5/1
  Divide_bc583/1 -> Subtract_104f5/2
  Add_a2f8c/1 -> Product_6c4da/2
  Constant_D_d3ce4/1 -> Product_66508/2
  Product_bf6fd/1 -> Product_be1f0/1
  State_T_m_SG_D_1_78758/1 -> Product_be1f0/2
  Constant_2.0_0911c/1 -> Product_fb956/1
  Constant_pi_fec9f/1 -> Product_fb956/2
  Product_6c4da/1 -> Divide_daabb/1
  Constant_x_qdd_bfa06/1 -> Divide_daabb/2
  Product_70d4f/1 -> Divide_5097b/1
  Constant_x_ddd_62384/1 -> Divide_5097b/2
  Product_66508/1 -> Product_ddd4f/1
  Product_be1f0/1 -> Product_045c9/1
  Constant_f0_398c2/1 -> Product_045c9/2
  Product_fb956/1 -> Product_00fef/1
  Constant_f0_221da/1 -> Product_00fef/2
  Divide_5097b/1 -> Add_45e48/2
  Product_ddd4f/1 -> Add_f78f9/1
  Product_045c9/1 -> Add_f78f9/2
  Product_00fef/1 -> Product_42e50/1
  Add_45e48/1 -> Product_42e50/2
  Add_f78f9/1 -> Subtract_42fe2/1
  Product_42e50/1 -> Subtract_42fe2/2
  Constant_2.0_7ed91/1 -> Product_93efb/1
  Constant_H_309df/1 -> Product_93efb/2
  Subtract_42fe2/1 -> Divide_180b6/1
  Product_93efb/1 -> Divide_180b6/2
  Divide_180b6/1 -> Blockout_d_w_SG_D_1_734e0/1

== system case6/SG_D_1/i_d_SG_D_1_block ==
  note: i_d_SG_D_1 in case6
      | $\frac{\sin\left(\theta _{\mathrm{SG},D,1}\right)\,\left(\frac{\psi _{\mathrm{1d},\mathrm{SG},D,1}\,\left(x_{\mathrm{dd}}-x_{\mathrm{ddd}}\right)}{x_{\mathrm{dd}}-x_{l}}-\psi _{d,\mathrm{SG},D,1}+\frac{\psi _{\mathrm{fd},\mathrm{SG},D,1}\,\left(x_{\mathrm{ddd}}-x_{l}\right)}{x_{\mathrm{dd}}-x_{l}}\right)}{x_{\mathrm{ddd}}}-\frac{\cos\left(\theta _{\mathrm{SG},D,1}\right)\,\left(\psi _{q,\mathrm{SG},D,1}+\frac{\psi _{\mathrm{gq},\mathrm{SG},D,1}\,\left(x_{l}-x_{\mathrm{qdd}}\right)}{x_{l}-x_{\mathrm{qd}}}+\frac{\psi _{\mathrm{kq},\mathrm{SG},D,1}\,\left(x_{\mathrm{qd}}-x_{\mathrm{qdd}}\right)}{x_{l}-x_{\mathrm{qd}}}\right)}{x_{\mathrm{qdd}}}$
      | Automatically generated on 2025-10-31 19:17:14 .
  State_psi_gq_SG_D_1_23547 : Inport
  State_psi_kq_SG_D_1_e0108 : Inport  Port=2
  State_psi_q_SG_D_1_a1fdb : Inport  Port=3
  State_theta_SG_D_1_3d426 : Inport  Port=4
  State_psi_1d_SG_D_1_bbdd2 : Inport  Port=5
  State_psi_d_SG_D_1_4d404 : Inport  Port=6
  State_psi_fd_SG_D_1_b7d62 : Inport  Port=7
  State_theta_SG_D_1_ed7ba : Inport  Port=8
  Add_0896f : Sum
  Add_3711e : Sum
  Add_3c211 : Sum
  Add_5abad : Sum
  Add_f934c : Sum
  Constant_-1_32ca5 : Constant  Value=-1
  Constant_-1_42e20 : Constant  Value=-1
  Constant_-1_42fb5 : Constant  Value=-1
  Constant_-1_5ffbe : Constant  Value=-1
  Constant_-1_c849e : Constant  Value=-1
  Constant_x_dd_0b643 : Constant  Value=x_dd
  Constant_x_dd_5489d : Constant  Value=x_dd
  Constant_x_dd_fc9bd : Constant  Value=x_dd
  Constant_x_ddd_6008a : Constant  Value=x_ddd
  Constant_x_ddd_74756 : Constant  Value=x_ddd
  Constant_x_ddd_9c611 : Constant  Value=x_ddd
  Constant_x_l_26e0b : Constant  Value=x_l
  Constant_x_l_30695 : Constant  Value=x_l
  Constant_x_l_3a68a : Constant  Value=x_l
  Constant_x_l_42f4f : Constant  Value=x_l
  Constant_x_l_b1d14 : Constant  Value=x_l
  Constant_x_l_cf378 : Constant  Value=x_l
  Constant_x_qd_064aa : Constant  Value=x_qd
  Constant_x_qd_5c461 : Constant  Value=x_qd
  Constant_x_qd_67469 : Constant  Value=x_qd
  Constant_x_qdd_5805d : Constant  Value=x_qdd
  Constant_x_qdd_884e6 : Constant  Value=x_qdd
  Constant_x_qdd_a370a : Constant  Value=x_qdd
  Divide_1cb78 : Product  Inputs=*/
  Divide_3b4c7 : Product  Inputs=*/
  Divide_8ff6d : Product  Inputs=*/
  Divide_c1231 : Product  Inputs=*/
  Divide_ecac2 : Product  Inputs=*/
  Divide_fca5d : Product  Inputs=*/
  MathFunc_cos_80118 : Trigonometry  Operator=cos
  MathFunc_sin_d1f11 : Trigonometry
  Product_31f7f : Product
  Product_3e36c : Product
  Product_669f4 : Product
  Product_7a9be : Product
  Product_99010 : Product
  Product_9cd82 : Product
  Product_b63aa : Product
  Product_d33e3 : Product
  Product_dab71 : Product
  Product_ea4ea : Product
  Product_f892e : Product
  Subtract_001ef : Sum  Inputs=+-
  Subtract_0abac : Sum  Inputs=+-
  Subtract_18bfe : Sum  Inputs=+-
  Subtract_19cf3 : Sum  Inputs=+-
  Subtract_230d1 : Sum  Inputs=+-
  Subtract_3df23 : Sum  Inputs=+-
  Subtract_73103 : Sum  Inputs=+-
  Subtract_ad33e : Sum  Inputs=+-
  Blockout_i_d_SG_D_1_69b6a : Outport
  wires:
  Constant_-1_42e20/1 -> Product_f892e/1
  Constant_x_l_30695/1 -> Product_f892e/2
  Constant_x_ddd_9c611/1 -> Subtract_73103/2
  Product_f892e/1 -> Add_0896f/1
  Constant_x_qdd_884e6/1 -> Subtract_ad33e/2
  Constant_x_l_cf378/1 -> Product_3e36c/2
  Constant_x_qd_064aa/1 -> Add_f934c/2
  Constant_x_qdd_5805d/1 -> Add_0896f/2
  Constant_x_qd_5c461/1 -> Subtract_ad33e/1
  MathFunc_cos_80118/1 -> Product_dab71/2
  Constant_-1_5ffbe/1 -> Product_3e36c/1
  Constant_-1_c849e/1 -> Product_99010/1
  Subtract_0abac/1 -> Blockout_i_d_SG_D_1_69b6a/1
  Constant_x_l_b1d14/1 -> Product_99010/2
  Divide_3b4c7/1 -> Subtract_3df23/1
  State_psi_gq_SG_D_1_23547/1 -> Product_669f4/1
  Subtract_230d1/1 -> Product_d33e3/2
  Add_0896f/1 -> Product_669f4/2
  Divide_8ff6d/1 -> Add_3c211/1
  Product_3e36c/1 -> Add_3711e/1
  Constant_x_qd_67469/1 -> Add_3711e/2
  State_psi_kq_SG_D_1_e0108/1 -> Product_ea4ea/1
  Add_3c211/1 -> Subtract_18bfe/1
  Add_3711e/1 -> Divide_3b4c7/2
  Subtract_ad33e/1 -> Product_ea4ea/2
  Product_99010/1 -> Add_f934c/1
  Constant_-1_42fb5/1 -> Product_b63aa/1
  State_psi_1d_SG_D_1_bbdd2/1 -> Product_b63aa/2
  Constant_x_dd_5489d/1 -> Subtract_73103/1
  Product_669f4/1 -> Divide_3b4c7/1
  Product_7a9be/1 -> Divide_fca5d/1
  Subtract_73103/1 -> Product_9cd82/2
  Product_ea4ea/1 -> Divide_1cb78/1
  Product_b63aa/1 -> Product_9cd82/1
  Add_f934c/1 -> Divide_1cb78/2
  Constant_x_dd_0b643/1 -> Subtract_001ef/1
  Subtract_3df23/1 -> Add_5abad/1
  Constant_x_l_42f4f/1 -> Subtract_001ef/2
  Constant_x_ddd_74756/1 -> Subtract_230d1/1
  Constant_x_l_26e0b/1 -> Subtract_230d1/2
  Divide_fca5d/1 -> Subtract_0abac/2
  Divide_1cb78/1 -> Subtract_3df23/2
  State_theta_SG_D_1_3d426/1 -> MathFunc_cos_80118/1
  Product_9cd82/1 -> Divide_8ff6d/1
  Subtract_001ef/1 -> Divide_8ff6d/2
  State_theta_SG_D_1_ed7ba/1 -> MathFunc_sin_d1f11/1
  State_psi_fd_SG_D_1_b7d62/1 -> Product_d33e3/1
  Constant_x_dd_fc9bd/1 -> Subtract_19cf3/1
  Constant_x_l_3a68a/1 -> Subtract_19cf3/2
  State_psi_q_SG_D_1_a1fdb/1 -> Add_5abad/2
  State_psi_d_SG_D_1_4d404/1 -> Add_3c211/2
  Constant_x_ddd_6008a/1 -> Divide_fca5d/2
  MathFunc_sin_d1f11/1 -> Product_7a9be/2
  Product_d33e3/1 -> Divide_c1231/1
  Constant_-1_32ca5/1 -> Product_31f7f/1
  Subtract_19cf3/1 -> Divide_c1231/2
  Add_5abad/1 -> Product_31f7f/2
  Divide_c1231/1 -> Subtract_18bfe/2
  Product_31f7f/1 -> Product_dab71/1
  Subtract_18bfe/1 -> Product_7a9be/1
  Constant_x_qdd_a370a/1 -> Divide_ecac2/2
  Product_dab71/1 -> Divide_ecac2/1
  Divide_ecac2/1 -> Subtract_0abac/1

== system case6/SG_D_1/i_q_SG_D_1_block ==
  note: i_q_SG_D_1 in case6
      | $-\frac{\sin\left(\theta _{\mathrm{SG},D,1}\right)\,\left(\psi _{q,\mathrm{SG},D,1}+\frac{\psi _{\mathrm{gq},\mathrm{SG},D,1}\,\left(x_{l}-x_{\mathrm{qdd}}\right)}{x_{l}-x_{\mathrm{qd}}}+\frac{\psi _{\mathrm{kq},\mathrm{SG},D,1}\,\left(x_{\mathrm{qd}}-x_{\mathrm{qdd}}\right)}{x_{l}-x_{\mathrm{qd}}}\right)}{x_{\mathrm{qdd}}}-\frac{\cos\left(\theta _{\mathrm{SG},D,1}\right)\,\left(\frac{\psi _{\mathrm{1d},\mathrm{SG},D,1}\,\left(x_{\mathrm{dd}}-x_{\mathrm{ddd}}\right)}{x_{\mathrm{dd}}-x_{l}}-\psi _{d,\mathrm{SG},D,1}+\frac{\psi _{\mathrm{fd},\mathrm{SG},D,1}\,\left(x_{\mathrm{ddd}}-x_{l}\right)}{x_{\mathrm{dd}}-x_{l}}\right)}{x_{\mathrm{ddd}}}$
      | Automatically generated on 2025-10-31 19:17:18 .
  State_psi_gq_SG_D_1_a3576 : Inport
  State_psi_kq_SG_D_1_a7435 : Inport  Port=2
  State_psi_q_SG_D_1_d8456 : Inport  Port=3
  State_theta_SG_D_1_21b86 : Inport  Port=4
  State_psi_1d_SG_D_1_a52dc : Inport  Port=5
  State_psi_d_SG_D_1_f2988 : Inport  Port=6
  State_psi_fd_SG_D_1_87227 : Inport  Port=7
  State_theta_SG_D_1_18b66 : Inport  Port=8
  Add_3e24d : Sum
  Add_b1598 : Sum
  Add_cc5f6 : Sum
  Add_e4304 : Sum
  Add_f0852 : Sum
  Add_f6086 : Sum
  Constant_-1_0a9e6 : Constant  Value=-1
  Constant_-1_231ae : Constant  Value=-1
  Constant_-1_d3e2d : Constant  Value=-1
  Constant_-1_e7917 : Constant  Value=-1
  Constant_-1_fded0 : Constant  Value=-1
  Constant_x_dd_5ed65 : Constant  Value=x_dd
  Constant_x_dd_62ea2 : Constant  Value=x_dd
  Constant_x_dd_8f0db : Constant  Value=x_dd
  Constant_x_ddd_92d3e : Constant  Value=x_ddd
  Constant_x_ddd_bf299 : Constant  Value=x_ddd
  Constant_x_ddd_d8039 : Constant  Value=x_ddd
  Constant_x_l_0e153 : Constant  Value=x_l
  Constant_x_l_2612f : Constant  Value=x_l
  Constant_x_l_2aa5d : Constant  Value=x_l
  Constant_x_l_80a55 : Constant  Value=x_l
  Constant_x_l_a99ac : Constant  Value=x_l
  Constant_x_l_ac33c : Constant  Value=x_l
  Constant_x_qd_0d638 : Constant  Value=x_qd
  Constant_x_qd_7c6d1 : Constant  Value=x_qd
  Constant_x_qd_9f68c : Constant  Value=x_qd
  Constant_x_qdd_67e63 : Constant  Value=x_qdd
  Constant_x_qdd_92ef3 : Constant  Value=x_qdd
  Constant_x_qdd_ec139 : Constant  Value=x_qdd
  Divide_269c9 : Product  Inputs=*/
  Divide_86666 : Product  Inputs=*/
  Divide_87c09 : Product  Inputs=*/
  Divide_933f2 : Product  Inputs=*/
  Divide_c5464 : Product  Inputs=*/
  Divide_e0f0c : Product  Inputs=*/
  MathFunc_cos_cbb38 : Trigonometry  Operator=cos
  MathFunc_sin_a810b : Trigonometry
  Product_0e395 : Product
  Product_1c62c : Product
  Product_61f91 : Product
  Product_6aba2 : Product
  Product_784ca : Product
  Product_7b53d : Product
  Product_9cb15 : Product
  Product_b11d4 : Product
  Product_d08b0 : Product
  Product_f5064 : Product
  Product_f9d24 : Product
  Subtract_18b76 : Sum  Inputs=+-
  Subtract_476a2 : Sum  Inputs=+-
  Subtract_5f27b : Sum  Inputs=+-
  Subtract_79d65 : Sum  Inputs=+-
  Subtract_838d2 : Sum  Inputs=+-
  Subtract_bde0a : Sum  Inputs=+-
  Subtract_f9ecb : Sum  Inputs=+-
  Blockout_i_q_SG_D_1_048b9 : Outport
  wires:
  State_theta_SG_D_1_18b66/1 -> MathFunc_cos_cbb38/1
  State_psi_fd_SG_D_1_87227/1 -> Product_1c62c/1
  Constant_-1_231ae/1 -> Product_0e395/1
  Constant_x_l_ac33c/1 -> Product_0e395/2
  Subtract_79d65/1 -> Product_1c62c/2
  Constant_x_l_a99ac/1 -> Subtract_18b76/2
  Product_0e395/1 -> Add_3e24d/1
  Constant_x_qdd_92ef3/1 -> Add_3e24d/2
  Constant_x_qd_9f68c/1 -> Subtract_476a2/1
  Constant_x_qdd_ec139/1 -> Divide_269c9/2
  MathFunc_sin_a810b/1 -> Product_784ca/2
  Constant_-1_e7917/1 -> Product_f5064/1
  Constant_x_qdd_67e63/1 -> Subtract_476a2/2
  Add_e4304/1 -> Product_d08b0/2
  Product_f9d24/1 -> Divide_e0f0c/1
  Constant_x_l_0e153/1 -> Product_f5064/2
  Constant_-1_fded0/1 -> Product_9cb15/1
  Constant_x_l_80a55/1 -> Product_9cb15/2
  State_psi_gq_SG_D_1_a3576/1 -> Product_f9d24/1
  Add_3e24d/1 -> Product_f9d24/2
  Divide_86666/1 -> Add_cc5f6/1
  Product_f5064/1 -> Add_b1598/1
  Divide_269c9/1 -> Add_f0852/1
  Constant_x_qd_7c6d1/1 -> Add_b1598/2
  State_psi_kq_SG_D_1_a7435/1 -> Product_7b53d/1
  Add_cc5f6/1 -> Subtract_5f27b/1
  Subtract_476a2/1 -> Product_7b53d/2
  Divide_e0f0c/1 -> Subtract_838d2/1
  Add_b1598/1 -> Divide_e0f0c/2
  Product_9cb15/1 -> Add_f6086/1
  Constant_x_qd_0d638/1 -> Add_f6086/2
  Constant_-1_0a9e6/1 -> Product_6aba2/1
  MathFunc_cos_cbb38/1 -> Product_61f91/2
  Product_1c62c/1 -> Divide_c5464/1
  State_psi_1d_SG_D_1_a52dc/1 -> Product_6aba2/2
  Constant_x_l_2612f/1 -> Subtract_bde0a/2
  Constant_x_dd_5ed65/1 -> Subtract_f9ecb/1
  Divide_c5464/1 -> Subtract_5f27b/2
  Constant_x_ddd_bf299/1 -> Subtract_f9ecb/2
  Product_61f91/1 -> Divide_87c09/1
  Product_7b53d/1 -> Divide_933f2/1
  Product_6aba2/1 -> Product_b11d4/1
  Add_f6086/1 -> Divide_933f2/2
  Subtract_f9ecb/1 -> Product_b11d4/2
  State_psi_d_SG_D_1_f2988/1 -> Add_cc5f6/2
  Constant_x_dd_62ea2/1 -> Subtract_18b76/1
  Constant_x_ddd_92d3e/1 -> Subtract_79d65/1
  Constant_x_l_2aa5d/1 -> Subtract_79d65/2
  Divide_87c09/1 -> Add_f0852/2
  Divide_933f2/1 -> Subtract_838d2/2
  State_theta_SG_D_1_21b86/1 -> MathFunc_sin_a810b/1
  Product_b11d4/1 -> Divide_86666/1
  Subtract_18b76/1 -> Divide_86666/2
  Constant_x_dd_8f0db/1 -> Subtract_bde0a/1
  Subtract_838d2/1 -> Add_e4304/1
  State_psi_q_SG_D_1_d8456/1 -> Add_e4304/2
  Subtract_bde0a/1 -> Divide_c5464/2
  Subtract_5f27b/1 -> Product_61f91/1
  Constant_-1_d3e2d/1 -> Product_d08b0/1
  Product_d08b0/1 -> Product_784ca/1
  Product_784ca/1 -> Divide_269c9/1
  Constant_x_ddd_d8039/1 -> Divide_87c09/2
  Add_f0852/1 -> Blockout_i_q_SG_D_1_048b9/1

== system case6/SG_D_1/theta_SG_D_1_out_block ==
  note: theta_SG_D_1_out in case6
      | $\theta _{\mathrm{SG},D,1}$
      | Automatically generated on 2025-10-31 19:17:20 .
  State_theta_SG_D_1_cf04f : Inport
  Blockout_theta_SG_D_1_out_53391 : Outport
  wires:
  State_theta_SG_D_1_cf04f/1 -> Blockout_theta_SG_D_1_out_53391/1

== system case6/SG_D_1/w_SG_D_1_out_block ==
  note: w_SG_D_1_out in case6
      | $w_{\mathrm{SG},D,1}$
      | Automatically generated on 2025-10-31 19:17:20 .
  State_w_SG_D_1_b0bc1 : Inport
  Blockout_w_SG_D_1_out_bc596 : Outport
  wires:
  State_w_SG_D_1_b0bc1/1 -> Blockout_w_SG_D_1_out_bc596/1
